simulink model "Just_Gas_Static"  (R2021a)
settings: Solver=ode23t  StartTime=0.0  StopTime=2  FixedStep=.001  MaxStep=0.01  RelTol=1e-3
libraries: fl_lib x11, nesl_utility x6
settings Model: Creator=se108102  LastModifiedBy=se108102
settings SolverCC: AlgebraicLoopSolver=TrustRegion
settings DebuggingCC: SFMachineParentedDataDiag=warning

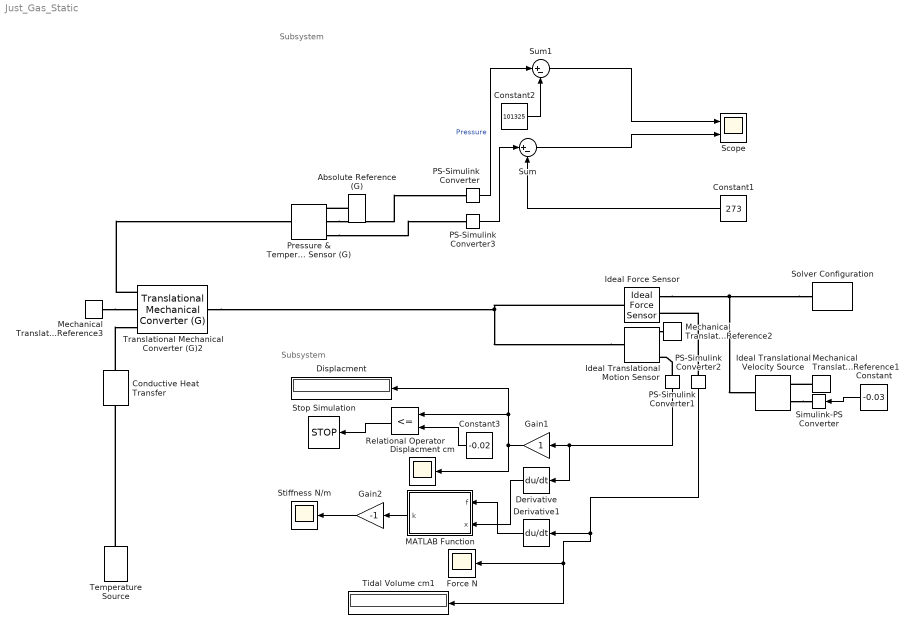
== system Just_Gas_Static ==
  note: Subsystem
  note: Subsystem
  Absolute Reference (G) : fl_lib/Gas/Elements/Absolute Reference (G)
      settings: SourceProductBaseCode=SS  InternalSimscapePortConfiguration="{\"Bottom\":[],\"Left\":[{\"id\":\"A\",\"label\":\"\",\"type\":\"foundation.gas.gas\"}],\"Right\":[],\"Top\":[]}"
  Conductive Heat Transfer : fl_lib/Thermal/Thermal Elements/Conductive Heat Transfer  area=200.96 cm^2  thickness=0.001 mm  th_cond=205 W/(m*K)  T_specify=off  T_priority=None  T=0 K  T_nominal_specify=off  T_nominal_unit=K  T_nominal_value=1  Q_specify=off  Q_priority=None  Q=0 W  Q_nominal_specify=off  Q_nominal_unit=W  Q_nominal_value=1
  Constant : Constant  Value=-0.03
  Constant1 : Constant  Value=273
  Constant2 : Constant  Value=101325
  Constant3 : Constant  Value=-0.02
  Derivative : Derivative
  Derivative1 : Derivative
  Displacment : Display
      settings: Decimation=5
  Displacment cm : Scope
  Force N : Scope
  Gain1 : Gain
  Gain2 : Gain  Gain=-1
  Ideal Force Sensor : fl_lib/Mechanical/Mechanical Sensors/Ideal Force Sensor
  Ideal Translational Motion Sensor : fl_lib/Mechanical/Mechanical Sensors/Ideal Translational Motion Sensor  offset=0 m
  Ideal Translational Velocity Source : fl_lib/Mechanical/Mechanical Sources/Ideal Translational Velocity Source
  MATLAB Function : MATLAB Function  TreatAsAtomicUnit=on
  Mechanical Translational Reference1 : fl_lib/Mechanical/Translational Elements/Mechanical Translational Reference
  Mechanical Translational Reference2 : fl_lib/Mechanical/Translational Elements/Mechanical Translational Reference
  Mechanical Translational Reference3 : fl_lib/Mechanical/Translational Elements/Mechanical Translational Reference
  PS-Simulink Converter : nesl_utility/PS-Simulink Converter  PhysicalDomain=network_engine_domain  SubClassName=ps_output  LeftPortType=input  RightPortType=output  PseudoPeriodic=off  Frequencies=[]  Unit=Pa  AffineConversion=off
      settings: SourceProductBaseCode=PW,SS
  PS-Simulink Converter1 : nesl_utility/PS-Simulink Converter  PhysicalDomain=network_engine_domain  SubClassName=ps_output  LeftPortType=input  RightPortType=output  PseudoPeriodic=off  Frequencies=[]  Unit=m  AffineConversion=off
      settings: SourceProductBaseCode=PW,SS
  PS-Simulink Converter2 : nesl_utility/PS-Simulink Converter  PhysicalDomain=network_engine_domain  SubClassName=ps_output  LeftPortType=input  RightPortType=output  PseudoPeriodic=off  Frequencies=[]  Unit=N  AffineConversion=off
      settings: SourceProductBaseCode=PW,SS
  PS-Simulink Converter3 : nesl_utility/PS-Simulink Converter  PhysicalDomain=network_engine_domain  SubClassName=ps_output  LeftPortType=input  RightPortType=output  PseudoPeriodic=off  Frequencies=[]  Unit=inherit  AffineConversion=off
      settings: SourceProductBaseCode=PW,SS
  Pressure & Temperature Sensor (G) : fl_lib/Gas/Sensors/Pressure & Temperature Sensor (G)
      settings: SourceProductBaseCode=SS  InternalSimscapePortConfiguration="{\"Bottom\":[],\"Left\":[{\"id\":\"A\",\"label\":\"A\",\"type\":\"foundation.gas.gas\"}],\"Right\":[{\"id\":\"B\",\"label\":\"B\",\"type\":\"foundation.gas.gas\"},{\"id\":\"P\",\"label\":\"P\",\"type\":\"output\"},{\"id\":\"T\",\"label\":\"T\",\"type\":\"output\"}],\"Top\":[]}"
  Relational Operator : RelationalOperator  Operator=<=  OutDataTypeStr=boolean  RndMeth=Simplest
  Scope : Scope  NumInputPorts=2
  Simulink-PS Converter : nesl_utility/Simulink-PS Converter  PhysicalDomain=network_engine_domain  SubClassName=ps_input  LeftPortType=input  RightPortType=output  PseudoPeriodic=off  Frequencies=[]  NoiseDistribution=none  NoiseParameters=[]  Unit=1  AffineConversion=off  FilteringAndDerivatives=provide  SimscapeFilterOrder=1  InputFilterTimeConstant=0.001  UdotUserProvided=0
      settings: SourceProductBaseCode=PW,SS
  Solver Configuration : nesl_utility/Solver Configuration  PhysicalDomain=network_engine_domain  SubClassName=solver  LeftPortType=input  RightPortType=generic  Tones=[]  Harmonics=[]  SimulateNoise=off  Profile=off  UseLocalSampling=off  EnableSwitchedLinearOptims=on  FrequencyDomain=off  UseCCode=off  RelTol=0.001  AbsTol=1e-06  MinStep=1e-09  ToWorkspace=off  RevertToSquareIcSolve=off  NumHomotopyIterations=100  PhasorMode=off  PhasorModeNumHarmonics=1  DoDC=off  ResidualTolerance=1e-09  UseLocalSolver=off  LocalSolverChoice=NE_BACKWARD_EULER_ADVANCER  LocalSolverSampleTime=0.001  DoFixedCost=off  MaxNonlinIter=3  MaxModeIter=2  ComputeImpulses=off  ImpulseIterations=2  LinearAlgebra=auto  EquationFormulation=NE_TIME_EF  DelaysMemoryBudget=1024  AutomaticFiltering=on  FilteringTimeConstant=0.001  PartitionStorageMethod=AS_NEEDED  PartitionMemoryBudget=1024  PartitionMethod=ROBUST
      settings: SourceProductBaseCode=PW,SS
  Stiffness N/m : Scope
  Stop Simulation : Stop
  Sum : Sum  Inputs=|+-
  Sum1 : Sum  Inputs=|+-
  Temperature Source : fl_lib/Thermal/Thermal Sources/Temperature Source  temperature=25 degC
  Tidal Volume cm1 : Display
      settings: Decimation=5
  Translational Mechanical Converter (G)2 : fl_lib/Gas/Elements/Translational Mechanical Converter (G)  mech_orientation=foundation.enum.MechOrientationTranslational.Positive  displacement_spec=foundation.enum.DisplacementSpec.Calculate  length_init=2 cm  interface_area=8.0384 cm^2  dead_volume=60 cm^3  area_A=7.06 mm^2  environment_spec=foundation.enum.pressure_spec.specified  environment_pressure=14.7 psi  p_I_specify=on  p_I_priority=High  p_I=14.7 psi  p_I_nominal_specify=off  p_I_nominal_unit=MPa  p_I_nominal_value=1  T_I_specify=on  T_I_priority=High  T_I=25 degC  T_I_nominal_specify=off  T_I_nominal_unit=K  T_I_nominal_value=1  rho_converter_specify=off  rho_converter_priority=None  rho_converter=1.2 kg/m^3  rho_converter_nominal_specify=off  rho_converter_nominal_unit=kg/m^3  rho_converter_nominal_value=1
      settings: SourceProductBaseCode=SS  InternalSimscapePortConfiguration="{\"Bottom\":[],\"Left\":[{\"id\":\"A\",\"label\":\"A\",\"type\":\"foundation.gas.gas\"},{\"id\":\"C\",\"label\":\"C\",\"type\":\"foundation.mechanical.translational.translational\"},{\"id\":\"H\",\"label\":\"H\",\"type\":\"foundation.thermal.thermal\"}],\"Right\":[{\"id\":\"R\",\"label\":\"R\",\"type\":\"foundation.mechanical.translational.translational\"}],\"Top\":[]}"
  wires:
  Constant/1 -> Simulink-PS Converter/1
  Gain1/1 -> Displacment/1, Relational Operator/1, Displacment cm/1
  MATLAB Function/1(k) -> Gain2/1
  Gain2/1 -> Stiffness N/m/1
  PS-Simulink Converter1/1 -> Derivative/1, Gain1/1
  PS-Simulink Converter2/1 -> Tidal Volume cm1/1, Force N/1, Derivative1/1
  Constant2/1 -> Sum1/2
  Sum1/1 -> Scope/1
  Constant1/1 -> Sum/2
  PS-Simulink Converter3/1 -> Sum/1
  Sum/1 -> Scope/2
  PS-Simulink Converter/1 -> Sum1/1  "Pressure"
  Relational Operator/1 -> Stop Simulation/1
  Constant3/1 -> Relational Operator/2
  Derivative/1 -> MATLAB Function/2(x)
  Derivative1/1 -> MATLAB Function/1(f)
  connections:
  Solver Configuration/RConn1 -- Ideal Force Sensor/RConn1 -- Ideal Translational Velocity Source/LConn1
  Ideal Translational Motion Sensor/LConn1 -- Ideal Force Sensor/LConn1 -- Translational Mechanical Converter (G)2/RConn1
  PS-Simulink Converter1/LConn1 -- Ideal Translational Motion Sensor/RConn3
  Ideal Translational Motion Sensor/RConn1 -- Mechanical Translational Reference2/LConn1
  PS-Simulink Converter2/LConn1 -- Ideal Force Sensor/RConn2
  Mechanical Translational Reference1/LConn1 -- Ideal Translational Velocity Source/RConn2
  Ideal Translational Velocity Source/RConn1 -- Simulink-PS Converter/RConn1
  Temperature Source/LConn1 -- Conductive Heat Transfer/RConn1
  Conductive Heat Transfer/LConn1 -- Translational Mechanical Converter (G)2/LConn3
  Mechanical Translational Reference3/LConn1 -- Translational Mechanical Converter (G)2/LConn2
  Translational Mechanical Converter (G)2/LConn1 -- Pressure & Temperature Sensor (G)/LConn1
  Pressure & Temperature Sensor (G)/RConn3 -- PS-Simulink Converter3/LConn1
  Absolute Reference (G)/LConn1 -- Pressure & Temperature Sensor (G)/RConn1
  Pressure & Temperature Sensor (G)/RConn2 -- PS-Simulink Converter/LConn1

== matlab function Just_Gas_Static/MATLAB Function ==
  data: f input; k output; x input
function k = fcn(f,x)

k = f/x;
